simulink model "sim_test"  (R2016a)
settings: Solver=ode3  StartTime=0.0  StopTime=Tsim  FixedStep=Ts  RelTol=1e-3
values from neighbouring files (symbols this model uses):
  dist = 1    [run_sim.m]
  P = ss(A,[Bw Bu],[Cz;Cy],[Dzw Dzu; Dyw zeros(1,1)])    [system_def.m]
  ref = 0    [run_sim.m]
  Tdist = 8    [run_sim.m]
  Tref = 2    [run_sim.m]
  x0 = [0;zeros(size(P.A,1)-1,1)]    [run_sim.m]
  xK0 = zeros(size(Ksys.A,1),1)    [run_sim.m]
undefined symbols (not defined in the file or in its folder): Ksys
settings Model: Creator=Matti  LastModifiedBy=Matti

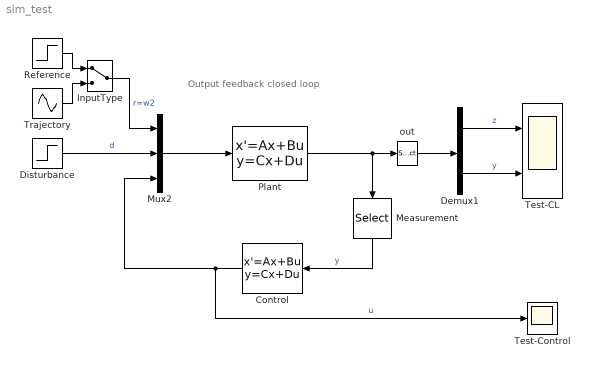
== system sim_test ==
  note: Output feedback closed loop
  Control : StateSpace  A=Ksys.A  B=Ksys.B  C=Ksys.C  D=Ksys.D  X0=xK0
  Demux1 : Demux  Outputs=2
  Disturbance : Step  Time=Tdist  After=dist  SampleTime=0
  InputType : ManualSwitch
  Measurement : Selector  InputPortWidth=3  IndexOptions=Index vector (dialog)  Indices=[3]  OutputSizes=1
  Mux2 : Mux  Inputs=3
  Plant : StateSpace  A=P.A  B=P.B  C=P.C  D=P.D  X0=x0
  Reference : Step  Time=Tref  After=ref  SampleTime=0
  Test-CL : Scope  NumInputPorts=2
  Test-Control : Scope
  Trajectory : Sin  Frequency=0.5  SampleTime=0
  out : Selector  InputPortWidth=3  IndexOptions=Index vector (dialog)  Indices=[1 3]  OutputSizes=1
  wires:
  Disturbance/1 -> Mux2/2  "d"
  Measurement/1 -> Control/1  "y"
  Plant/1 -> Measurement/1, out/1
  Control/1 -> Test-Control/1, Mux2/3  "u"
  Demux1/2 -> Test-CL/2  "y"
  Mux2/1 -> Plant/1
  Reference/1 -> InputType/1
  InputType/1 -> Mux2/1  "r=w2"
  Trajectory/1 -> InputType/2
  Demux1/1 -> Test-CL/1  "z"
  out/1 -> Demux1/1
